simulink model "frequencyResp"  (R2018a)
settings: Solver=ode45  StartTime=0.0  StopTime=2  RelTol=1e-7
settings Model: Creator=ewk15101  LastModifiedBy=ewk15101

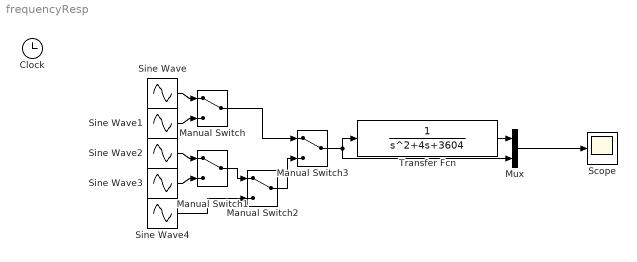
== system frequencyResp ==
  Clock : Clock
  Manual Switch{,1..3} (4 alike) : ManualSwitch
  Mux : Mux  Inputs=2
  Scope : Scope
  Sine Wave : Sin  Frequency=20  SampleTime=0
  Sine Wave1 : Sin  Frequency=50  SampleTime=0
  Sine Wave2 : Sin  Frequency=60  SampleTime=0
  Sine Wave3 : Sin  Frequency=80  SampleTime=0
  Sine Wave4 : Sin  Frequency=110  SampleTime=0
  Transfer Fcn : TransferFcn  Denominator=[1 4 3604]
  wires:
  Transfer Fcn/1 -> Mux/1
  Mux/1 -> Scope/1
  Sine Wave/1 -> Manual Switch/1
  Sine Wave1/1 -> Manual Switch/2
  Sine Wave2/1 -> Manual Switch1/1
  Sine Wave3/1 -> Manual Switch1/2
  Manual Switch1/1 -> Manual Switch2/1
  Sine Wave4/1 -> Manual Switch2/2
  Manual Switch/1 -> Manual Switch3/1
  Manual Switch2/1 -> Manual Switch3/2
  Manual Switch3/1 -> Mux/2, Transfer Fcn/1
